simulink model "MPC_model_complete"  (R2021a)
settings: Solver=FixedStepAuto  StartTime=0.0  StopTime=3  FixedStep=0.01  RelTol=1e-3
settings Model: Creator=Shayan  LastModifiedBy=SHAMBHAVI
settings SolverCC: AlgebraicLoopSolver=TrustRegion
settings DataIOCC: ReturnWorkspaceOutputs=off
settings OptimizationCC: LifeSpan=inf
settings DebuggingCC: SFMachineParentedDataDiag=warning  ArithmeticOperatorsInVariantConditions=warning
settings SFSimCC: CustomCodeUndefinedFunction=UseInterfaceOnly
settings CodeAppCC: StateflowObjectComments=on

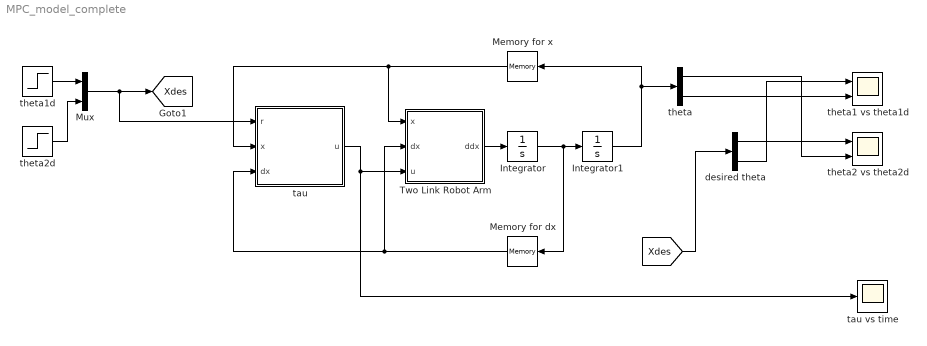
== system MPC_model_complete ==
  Integrator : Integrator  InitialCondition=[0 0]
  Integrator1 : Integrator  InitialCondition=[pi/2 -pi/2]
  Memory for dx : Memory  InitialCondition=[0 0]
  Memory for x : Memory  InitialCondition=[pi/2 -pi/2]
  Mux : Mux  Inputs=2
  Two Link Robot Arm : MATLAB Function  TreatAsAtomicUnit=on
  desired theta : Demux  Outputs=2
  tau : MATLAB Function  TreatAsAtomicUnit=on
  tau vs time : Scope
  theta : Demux  Outputs=2
  theta1 vs theta1d : Scope  NumInputPorts=2
  theta1d : Step  Time=0  After=0  SampleTime=0
  theta2 vs theta2d : Scope  NumInputPorts=2
  theta2d : Step  Time=0  After=0  SampleTime=0
  tag scope: Xdes=global
  wires:
  Integrator/1 -> Integrator1/1, Memory for dx/1
  Two Link Robot Arm/1(ddx) -> Integrator/1
  theta1d/1 -> Mux/1
  theta2d/1 -> Mux/2
  [Xdes] -> desired theta/1
  Integrator1/1 -> Memory for x/1, theta/1
  desired theta/1 -> theta2 vs theta2d/1
  theta/1 -> theta2 vs theta2d/2
  theta/2 -> theta1 vs theta1d/2
  desired theta/2 -> theta1 vs theta1d/1
  Memory for dx/1 -> tau/3(dx), Two Link Robot Arm/2(dx)
  tau/1(u) -> tau vs time/1, Two Link Robot Arm/3(u)
  Memory for x/1 -> tau/2(x), Two Link Robot Arm/1(x)
  Mux/1 -> tau/1(r), [Xdes]

== matlab function MPC_model_complete/Two Link Robot Arm ==
  data: x input; dx input; u input; ddx output
function ddx = fcn(x,dx,u)

M1 = 1;
M2 = 1;
L1 = 1;
L2 = 1;
g = 9.81;
G = [-(M1+M2)*g*L1-M2*g*L2*sin(x(1)+x(2));...
    -M2*g*L2*sin(x(1)+x(2));];
C = [M1*L1*L2*(2*dx(1)*dx(2) + dx(1)^2)*sin(x(2));...
    -M2*L1*L2*dx(1)*dx(2)*sin(x(2));];
M = [-(M1+M2)*L1^2 + M2*L2^2 + 2*M2*L1*L2*cos(x(2)), M2*L2^2 + M2*L1*L2*cos(x(2));...
     M2*L2^2 + M2*L1*L2*cos(x(2)),  M2*L2^2;];
ddx = inv(M)*(-C-G+u);

== matlab function MPC_model_complete/tau ==
  data: r input; u output; x input; dx input
function u  = fcn(r,x,dx)
%r is the reference angle r(1) = -pi/3 and r(2)=pi/3
k1 = 15.99;
k2 = 5.65;
k3 = k1;
v = [k3*r(1) - k1*x(1) - k2*dx(1);...
     (k3*r(2) - k1*x(2) - k2*dx(2));];
M1 = 1;
M2 = 1;
L1 = 1;
L2 = 1;
g = 9.81;
G = [-(M1+M2)*g*L1-M2*g*L2*sin(x(1)+x(2));...
    -M2*g*L2*sin(x(1)+x(2));]; %gravitational 
C = [M1*L1*L2*(2*dx(1)*dx(2) + dx(1)^2)*sin(x(2));...
    -M2*L1*L2*dx(1)*dx(2)*sin(x(2));]; %coriolis
M = [-(M1+M2)*L1^2 + M2*L2^2 + 2*M2*L1*L2*cos(x(2)), M2*L2^2 + M2*L1*L2*cos(x(2));...
     M2*L2^2 + M2*L1*L2*cos(x(2)),  M2*L2^2;]; %intertial component

u = M*v + C + G; %two dimensional tau vector coloumn matrix
